simulink model "labFinal_3"  (R2018b)
settings: Solver=FixedStepDiscrete  StartTime=0.0  StopTime=10.0  FixedStep=1  RelTol=1e-3
libraries: hdlsllib x17
(part 1 of 2)
settings Model: Creator=mllax8  LastModifiedBy=mllax8

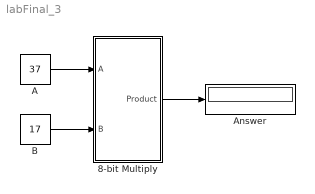
== system labFinal_3 ==
  8-bit Multiply : Subsystem
  A : Constant  Value=37  OutDataTypeStr=uint8  SampleTime=1
  Answer : Display
  B : Constant  Value=17  OutDataTypeStr=uint8  SampleTime=1
  wires:
  B/1 -> 8-bit Multiply/2(B)
  A/1 -> 8-bit Multiply/1(A)
  8-bit Multiply/1(Product) -> Answer/1

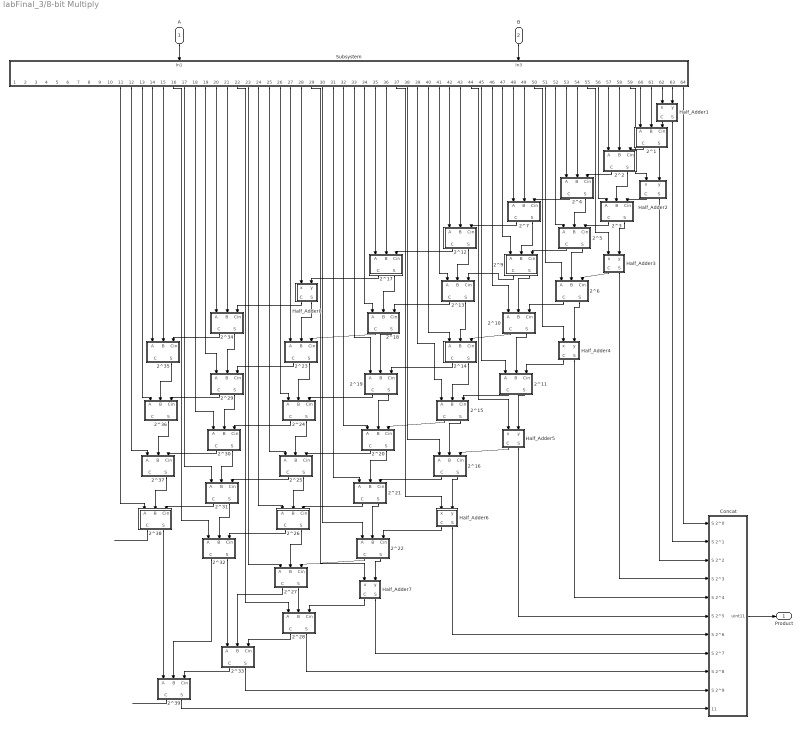
== system labFinal_3/8-bit Multiply ==
  A : Inport  OutDataTypeStr=uint8
  B : Inport  Port=2  OutDataTypeStr=uint8
  2^1 : Subsystem
  2^10 : Subsystem
  2^11 : Subsystem
  2^12 : Subsystem
  2^13 : Subsystem
  2^14 : Subsystem
  2^15 : Subsystem
  2^16 : Subsystem
  2^17 : Subsystem
  2^18 : Subsystem
  2^19 : Subsystem
  2^2 : Subsystem
  2^20 : Subsystem
  2^21 : Subsystem
  2^22 : Subsystem
  2^23 : Subsystem
  2^24 : Subsystem
  2^25 : Subsystem
  2^26 : Subsystem
  2^27 : Subsystem
  2^28 : Subsystem
  2^29 : Subsystem
  2^3 : Subsystem
  2^30 : Subsystem
  2^31 : Subsystem
  2^32 : Subsystem
  2^33 : Subsystem
  2^34 : Subsystem
  2^35 : Subsystem
  2^36 : Subsystem
  2^37 : Subsystem
  2^38 : Subsystem
  2^39 : Subsystem
  2^4 : Subsystem
  2^5 : Subsystem
  2^6 : Subsystem
  2^7 : Subsystem
  2^9 : Subsystem
  Concat : Subsystem
  Half_Adder1 : Subsystem
  Half_Adder2 : Subsystem
  Half_Adder3 : Subsystem
  Half_Adder4 : Subsystem
  Half_Adder5 : Subsystem
  Half_Adder6 : Subsystem
  Half_Adder7 : Subsystem
  Half_Adder8 : Subsystem
  Subsystem : Subsystem
  Product : Outport
  wires:
  A/1 -> Subsystem/1(In1)
  B/1 -> Subsystem/2(In3)
  Subsystem/63(A0B1) -> Half_Adder1/2(y)
  Subsystem/62(A1B0) -> Half_Adder1/1(x)
  Half_Adder1/1(C) -> 2^1/3(Cin)
  Subsystem/61(A1B1) -> 2^1/2(B)
  Subsystem/60(A0B2) -> 2^1/1(A)
  Subsystem/59(A2B0) -> Half_Adder2/1(x)
  2^1/2(S) -> Half_Adder2/2(y)
  2^1/1(C) -> 2^2/3(Cin)
  Subsystem/58(A0B3) -> 2^2/2(B)
  Subsystem/57(A1B2) -> 2^2/1(A)
  Half_Adder2/1(C) -> 2^3/3(Cin)
  2^2/2(S) -> 2^3/2(B)
  Subsystem/56(A2B1) -> 2^3/1(A)
  2^3/1(C) -> 2^5/3(Cin)
  Subsystem/55(A3B0) -> Half_Adder3/1(x)
  2^3/2(S) -> Half_Adder3/2(y)
  Subsystem/54(A0B4) -> 2^4/2(B)
  Subsystem/53(A1B3) -> 2^4/1(A)
  2^2/1(C) -> 2^4/3(Cin)
  2^4/1(C) -> 2^7/3(Cin)
  2^4/2(S) -> 2^5/2(B)
  Subsystem/52(A2B2) -> 2^5/1(A)
  2^5/1(C) -> 2^9/3(Cin)
  Half_Adder3/1(C) -> 2^6/3(Cin)
  2^5/2(S) -> 2^6/2(B)
  Subsystem/51(A3B1) -> 2^6/1(A)
  2^6/1(C) -> 2^10/3(Cin)
  2^6/2(S) -> Half_Adder4/2(y)
  Subsystem/50(A4B0) -> Half_Adder4/1(x)
  Half_Adder4/1(C) -> 2^11/3(Cin)
  Subsystem/49(A0B5) -> 2^7/2(B)
  Subsystem/48(A1B4) -> 2^7/1(A)
  Subsystem/47(A2B3) -> 2^9/1(A)
  2^9/2(S) -> 2^10/2(B)
  2^9/1(C) -> 2^13/3(Cin)
  2^7/2(S) -> 2^9/2(B)
  2^7/1(C) -> 2^12/3(Cin)
  Subsystem/46(A3B2) -> 2^10/1(A)
  2^10/1(C) -> 2^14/3(Cin)
  2^10/2(S) -> 2^11/2(B)
  Half_Adder3/2(S) -> Concat/4(S 2^3)
  Half_Adder4/2(S) -> Concat/5(S 2^4)
  2^11/1(C) -> 2^15/3(Cin)
  Subsystem/44(A5B0) -> Half_Adder5/1(x)
  2^11/2(S) -> Half_Adder5/2(y)
  Half_Adder5/2(S) -> Concat/6(S 2^5)
  Half_Adder5/1(C) -> 2^16/3(Cin)
  Subsystem/43(A0B6) -> 2^12/2(B)
  Subsystem/42(A1B5) -> 2^12/1(A)
  2^12/2(S) -> 2^13/2(B)
  Subsystem/41(A2B4) -> 2^13/1(A)
  Subsystem/45(A4B1) -> 2^11/1(A)
  2^13/1(C) -> 2^18/3(Cin)
  2^13/2(S) -> 2^14/2(B)
  Subsystem/40(A3B3) -> 2^14/1(A)
  2^14/2(S) -> 2^15/2(B)
  Subsystem/39(A4B2) -> 2^15/1(A)
  2^15/2(S) -> 2^16/2(B)
  Subsystem/38(A5B1) -> 2^16/1(A)
  2^15/1(C) -> 2^20/3(Cin)
  2^16/1(C) -> 2^21/3(Cin)
  Subsystem/37(A6B0) -> Half_Adder6/1(x)
  2^16/2(S) -> Half_Adder6/2(y)
  Half_Adder6/2(S) -> Concat/7(S 2^6)
  Half_Adder6/1(C) -> 2^22/3(Cin)
  2^17/1(C) -> Half_Adder8/2(y)
  2^12/1(C) -> 2^17/3(Cin)
  2^18/2(S) -> 2^19/2(B)
  2^21/1(C) -> 2^26/3(Cin)
  Subsystem/33(A3B4) -> 2^19/1(A)
  2^19/2(S) -> 2^20/2(B)
  Subsystem/34(A2B5) -> 2^18/1(A)
  Subsystem/32(A4B3) -> 2^20/1(A)
  2^20/2(S) -> 2^21/2(B)
  2^18/1(C) -> 2^23/3(Cin)
  Subsystem/31(A5B2) -> 2^21/1(A)
  2^17/2(S) -> 2^18/2(B)
  Subsystem/36(A0B7) -> 2^17/2(B)
  Subsystem/35(A1B6) -> 2^17/1(A)
  2^14/1(C) -> 2^19/3(Cin)
  2^21/2(S) -> 2^22/2(B)
  Subsystem/30(A6B1) -> 2^22/1(A)
  Subsystem/64(A0B0) -> Concat/1(S 2^0)
  Half_Adder2/2(S) -> Concat/3(S 2^2)
  2^22/2(S) -> Half_Adder7/2(y)
  Subsystem/29(A7B0) -> Half_Adder7/1(x)
  Subsystem/28(A1B7) -> Half_Adder8/1(x)
  Subsystem/27(A2B6) -> 2^23/1(A)
  Half_Adder8/2(S) -> 2^23/2(B)
  Half_Adder8/1(C) -> 2^34/3(Cin)
  2^19/1(C) -> 2^24/3(Cin)
  2^23/2(S) -> 2^24/2(B)
  Subsystem/26(A3B5) -> 2^24/1(A)
  2^20/1(C) -> 2^25/3(Cin)
  2^24/2(S) -> 2^25/2(B)
  Subsystem/25(A4B4) -> 2^25/1(A)
  2^24/1(C) -> 2^30/3(Cin)
  2^25/2(S) -> 2^26/2(B)
  2^25/1(C) -> 2^31/3(Cin)
  2^22/1(C) -> 2^27/3(Cin)
  Subsystem/24(A5B3) -> 2^26/1(A)
  Subsystem/23(A6B2) -> 2^27/1(A)
  Subsystem/22(A7B1) -> 2^28/1(A)
  2^26/2(S) -> 2^27/2(B)
  Half_Adder7/1(C) -> 2^28/3(Cin)
  2^27/2(S) -> 2^28/2(B)
  2^26/1(C) -> 2^32/3(Cin)
  Half_Adder7/2(S) -> Concat/8(S 2^7)
  2^28/1(C) -> 2^33/3(Cin)
  2^28/2(S) -> Concat/9(S 2^8)
  2^29/2(S) -> 2^30/2(B)
  2^30/2(S) -> 2^31/2(B)
  2^31/2(S) -> 2^32/2(B)
  Subsystem/21(A2B7) -> 2^34/2(B)
  Subsystem/20(A3B6) -> 2^34/1(A)
  2^23/1(C) -> 2^29/3(Cin)
  2^34/2(S) -> 2^29/2(B)
  Subsystem/19(A4B5) -> 2^29/1(A)
  Subsystem/18(A5B4) -> 2^30/1(A)
  Subsystem/17(A6B3) -> 2^31/1(A)
  Subsystem/16(A7B2) -> 2^32/1(A)
  2^32/2(S) -> 2^33/1(A)
  2^27/1(C) -> 2^33/2(B)
  2^33/2(S) -> Concat/10(S 2^9)
  2^32/1(C) -> 2^39/2(B)
  2^33/1(C) -> 2^39/3(Cin)
  2^34/1(C) -> 2^35/3(Cin)
  Subsystem/15(A3B7) -> 2^35/2(B)
  Subsystem/14(A4B6) -> 2^35/1(A)
  2^35/2(S) -> 2^36/2(B)
  2^29/1(C) -> 2^36/3(Cin)
  2^30/1(C) -> 2^37/3(Cin)
  2^36/2(S) -> 2^37/2(B)
  Subsystem/13(A5B5) -> 2^36/1(A)
  Subsystem/12(A6B4) -> 2^37/1(A)
  Subsystem/11(A7B3) -> 2^38/1(A)
  2^31/1(C) -> 2^38/3(Cin)
  2^37/2(S) -> 2^38/2(B)
  2^38/2(S) -> 2^39/1(A)
  2^38/1(C) -> ?
  2^39/1(C) -> ?
  2^39/2(S) -> Concat/11(S 2^10)
  Half_Adder1/2(S) -> Concat/2(S 2^1)
  Concat/1(uint11) -> Product/1

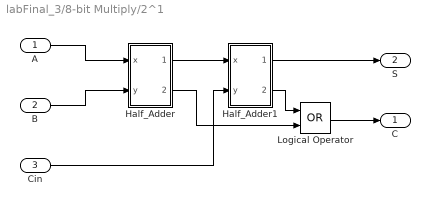
== system labFinal_3/8-bit Multiply/2^1 ==
  A : Inport
  B : Inport  Port=2
  Cin : Inport  Port=3
  Half_Adder : Subsystem
  Half_Adder1 : Subsystem
  Logical Operator : Logic  Operator=OR  AllPortsSameDT=off  OutDataTypeStr=boolean
  C : Outport
  S : Outport  Port=2
  wires:
  Half_Adder1/1(Sum) -> S/1
  Cin/1 -> Half_Adder1/2(y)
  Logical Operator/1 -> C/1
  Half_Adder1/2(Carry) -> Logical Operator/1
  A/1 -> Half_Adder/1(x)
  B/1 -> Half_Adder/2(y)
  Half_Adder/2(Carry) -> Logical Operator/2
  Half_Adder/1(Sum) -> Half_Adder1/1(x)

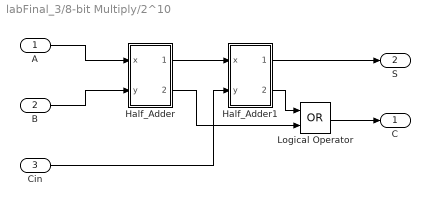
== system labFinal_3/8-bit Multiply/2^10 ==
  A : Inport
  B : Inport  Port=2
  Cin : Inport  Port=3
  Half_Adder : Subsystem
  Half_Adder1 : Subsystem
  Logical Operator : Logic  Operator=OR  AllPortsSameDT=off  OutDataTypeStr=boolean
  C : Outport
  S : Outport  Port=2
  wires:
  Half_Adder1/1(Sum) -> S/1
  Cin/1 -> Half_Adder1/2(y)
  Logical Operator/1 -> C/1
  Half_Adder1/2(Carry) -> Logical Operator/1
  A/1 -> Half_Adder/1(x)
  B/1 -> Half_Adder/2(y)
  Half_Adder/2(Carry) -> Logical Operator/2
  Half_Adder/1(Sum) -> Half_Adder1/1(x)

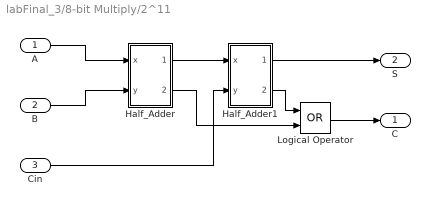
== system labFinal_3/8-bit Multiply/2^11 ==
  A : Inport
  B : Inport  Port=2
  Cin : Inport  Port=3
  Half_Adder : Subsystem
  Half_Adder1 : Subsystem
  Logical Operator : Logic  Operator=OR  AllPortsSameDT=off  OutDataTypeStr=boolean
  C : Outport
  S : Outport  Port=2
  wires:
  Half_Adder1/1(Sum) -> S/1
  Cin/1 -> Half_Adder1/2(y)
  Logical Operator/1 -> C/1
  Half_Adder1/2(Carry) -> Logical Operator/1
  A/1 -> Half_Adder/1(x)
  B/1 -> Half_Adder/2(y)
  Half_Adder/2(Carry) -> Logical Operator/2
  Half_Adder/1(Sum) -> Half_Adder1/1(x)

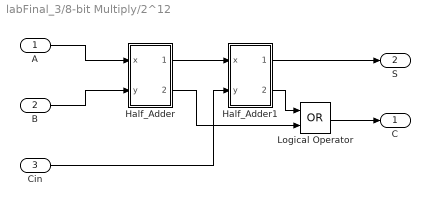
== system labFinal_3/8-bit Multiply/2^12 ==
  A : Inport
  B : Inport  Port=2
  Cin : Inport  Port=3
  Half_Adder : Subsystem
  Half_Adder1 : Subsystem
  Logical Operator : Logic  Operator=OR  AllPortsSameDT=off  OutDataTypeStr=boolean
  C : Outport
  S : Outport  Port=2
  wires:
  Half_Adder1/1(Sum) -> S/1
  Cin/1 -> Half_Adder1/2(y)
  Logical Operator/1 -> C/1
  Half_Adder1/2(Carry) -> Logical Operator/1
  A/1 -> Half_Adder/1(x)
  B/1 -> Half_Adder/2(y)
  Half_Adder/2(Carry) -> Logical Operator/2
  Half_Adder/1(Sum) -> Half_Adder1/1(x)

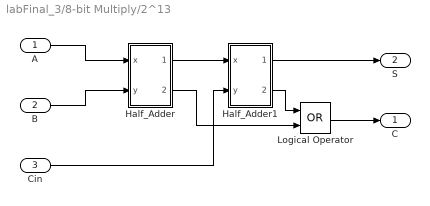
== system labFinal_3/8-bit Multiply/2^13 ==
  A : Inport
  B : Inport  Port=2
  Cin : Inport  Port=3
  Half_Adder : Subsystem
  Half_Adder1 : Subsystem
  Logical Operator : Logic  Operator=OR  AllPortsSameDT=off  OutDataTypeStr=boolean
  C : Outport
  S : Outport  Port=2
  wires:
  Half_Adder1/1(Sum) -> S/1
  Cin/1 -> Half_Adder1/2(y)
  Logical Operator/1 -> C/1
  Half_Adder1/2(Carry) -> Logical Operator/1
  A/1 -> Half_Adder/1(x)
  B/1 -> Half_Adder/2(y)
  Half_Adder/2(Carry) -> Logical Operator/2
  Half_Adder/1(Sum) -> Half_Adder1/1(x)

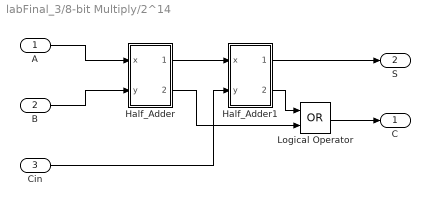
== system labFinal_3/8-bit Multiply/2^14 ==
  A : Inport
  B : Inport  Port=2
  Cin : Inport  Port=3
  Half_Adder : Subsystem
  Half_Adder1 : Subsystem
  Logical Operator : Logic  Operator=OR  AllPortsSameDT=off  OutDataTypeStr=boolean
  C : Outport
  S : Outport  Port=2
  wires:
  Half_Adder1/1(Sum) -> S/1
  Cin/1 -> Half_Adder1/2(y)
  Logical Operator/1 -> C/1
  Half_Adder1/2(Carry) -> Logical Operator/1
  A/1 -> Half_Adder/1(x)
  B/1 -> Half_Adder/2(y)
  Half_Adder/2(Carry) -> Logical Operator/2
  Half_Adder/1(Sum) -> Half_Adder1/1(x)

== system labFinal_3/8-bit Multiply/2^15 ==
  A : Inport
  B : Inport  Port=2
  Cin : Inport  Port=3
  Half_Adder : Subsystem
  Half_Adder1 : Subsystem
  Logical Operator : Logic  Operator=OR  AllPortsSameDT=off  OutDataTypeStr=boolean
  C : Outport
  S : Outport  Port=2
  wires:
  Half_Adder1/1(Sum) -> S/1
  Cin/1 -> Half_Adder1/2(y)
  Logical Operator/1 -> C/1
  Half_Adder1/2(Carry) -> Logical Operator/1
  A/1 -> Half_Adder/1(x)
  B/1 -> Half_Adder/2(y)
  Half_Adder/2(Carry) -> Logical Operator/2
  Half_Adder/1(Sum) -> Half_Adder1/1(x)

== system labFinal_3/8-bit Multiply/2^16 ==
  A : Inport
  B : Inport  Port=2
  Cin : Inport  Port=3
  Half_Adder : Subsystem
  Half_Adder1 : Subsystem
  Logical Operator : Logic  Operator=OR  AllPortsSameDT=off  OutDataTypeStr=boolean
  C : Outport
  S : Outport  Port=2
  wires:
  Half_Adder1/1(Sum) -> S/1
  Cin/1 -> Half_Adder1/2(y)
  Logical Operator/1 -> C/1
  Half_Adder1/2(Carry) -> Logical Operator/1
  A/1 -> Half_Adder/1(x)
  B/1 -> Half_Adder/2(y)
  Half_Adder/2(Carry) -> Logical Operator/2
  Half_Adder/1(Sum) -> Half_Adder1/1(x)

== system labFinal_3/8-bit Multiply/2^17 ==
  A : Inport
  B : Inport  Port=2
  Cin : Inport  Port=3
  Half_Adder : Subsystem
  Half_Adder1 : Subsystem
  Logical Operator : Logic  Operator=OR  AllPortsSameDT=off  OutDataTypeStr=boolean
  C : Outport
  S : Outport  Port=2
  wires:
  Half_Adder1/1(Sum) -> S/1
  Cin/1 -> Half_Adder1/2(y)
  Logical Operator/1 -> C/1
  Half_Adder1/2(Carry) -> Logical Operator/1
  A/1 -> Half_Adder/1(x)
  B/1 -> Half_Adder/2(y)
  Half_Adder/2(Carry) -> Logical Operator/2
  Half_Adder/1(Sum) -> Half_Adder1/1(x)

== system labFinal_3/8-bit Multiply/2^18 ==
  A : Inport
  B : Inport  Port=2
  Cin : Inport  Port=3
  Half_Adder : Subsystem
  Half_Adder1 : Subsystem
  Logical Operator : Logic  Operator=OR  AllPortsSameDT=off  OutDataTypeStr=boolean
  C : Outport
  S : Outport  Port=2
  wires:
  Half_Adder1/1(Sum) -> S/1
  Cin/1 -> Half_Adder1/2(y)
  Logical Operator/1 -> C/1
  Half_Adder1/2(Carry) -> Logical Operator/1
  A/1 -> Half_Adder/1(x)
  B/1 -> Half_Adder/2(y)
  Half_Adder/2(Carry) -> Logical Operator/2
  Half_Adder/1(Sum) -> Half_Adder1/1(x)

== system labFinal_3/8-bit Multiply/2^19 ==
  A : Inport
  B : Inport  Port=2
  Cin : Inport  Port=3
  Half_Adder : Subsystem
  Half_Adder1 : Subsystem
  Logical Operator : Logic  Operator=OR  AllPortsSameDT=off  OutDataTypeStr=boolean
  C : Outport
  S : Outport  Port=2
  wires:
  Half_Adder1/1(Sum) -> S/1
  Cin/1 -> Half_Adder1/2(y)
  Logical Operator/1 -> C/1
  Half_Adder1/2(Carry) -> Logical Operator/1
  A/1 -> Half_Adder/1(x)
  B/1 -> Half_Adder/2(y)
  Half_Adder/2(Carry) -> Logical Operator/2
  Half_Adder/1(Sum) -> Half_Adder1/1(x)

== system labFinal_3/8-bit Multiply/2^2 ==
  A : Inport
  B : Inport  Port=2
  Cin : Inport  Port=3
  Half_Adder : Subsystem
  Half_Adder1 : Subsystem
  Logical Operator : Logic  Operator=OR  AllPortsSameDT=off  OutDataTypeStr=boolean
  C : Outport
  S : Outport  Port=2
  wires:
  Half_Adder1/1(Sum) -> S/1
  Cin/1 -> Half_Adder1/2(y)
  Logical Operator/1 -> C/1
  Half_Adder1/2(Carry) -> Logical Operator/1
  A/1 -> Half_Adder/1(x)
  B/1 -> Half_Adder/2(y)
  Half_Adder/2(Carry) -> Logical Operator/2
  Half_Adder/1(Sum) -> Half_Adder1/1(x)

== system labFinal_3/8-bit Multiply/2^20 ==
  A : Inport
  B : Inport  Port=2
  Cin : Inport  Port=3
  Half_Adder : Subsystem
  Half_Adder1 : Subsystem
  Logical Operator : Logic  Operator=OR  AllPortsSameDT=off  OutDataTypeStr=boolean
  C : Outport
  S : Outport  Port=2
  wires:
  Half_Adder1/1(Sum) -> S/1
  Cin/1 -> Half_Adder1/2(y)
  Logical Operator/1 -> C/1
  Half_Adder1/2(Carry) -> Logical Operator/1
  A/1 -> Half_Adder/1(x)
  B/1 -> Half_Adder/2(y)
  Half_Adder/2(Carry) -> Logical Operator/2
  Half_Adder/1(Sum) -> Half_Adder1/1(x)

== system labFinal_3/8-bit Multiply/2^21 ==
  A : Inport
  B : Inport  Port=2
  Cin : Inport  Port=3
  Half_Adder : Subsystem
  Half_Adder1 : Subsystem
  Logical Operator : Logic  Operator=OR  AllPortsSameDT=off  OutDataTypeStr=boolean
  C : Outport
  S : Outport  Port=2
  wires:
  Half_Adder1/1(Sum) -> S/1
  Cin/1 -> Half_Adder1/2(y)
  Logical Operator/1 -> C/1
  Half_Adder1/2(Carry) -> Logical Operator/1
  A/1 -> Half_Adder/1(x)
  B/1 -> Half_Adder/2(y)
  Half_Adder/2(Carry) -> Logical Operator/2
  Half_Adder/1(Sum) -> Half_Adder1/1(x)

== system labFinal_3/8-bit Multiply/2^22 ==
  A : Inport
  B : Inport  Port=2
  Cin : Inport  Port=3
  Half_Adder : Subsystem
  Half_Adder1 : Subsystem
  Logical Operator : Logic  Operator=OR  AllPortsSameDT=off  OutDataTypeStr=boolean
  C : Outport
  S : Outport  Port=2
  wires:
  Half_Adder1/1(Sum) -> S/1
  Cin/1 -> Half_Adder1/2(y)
  Logical Operator/1 -> C/1
  Half_Adder1/2(Carry) -> Logical Operator/1
  A/1 -> Half_Adder/1(x)
  B/1 -> Half_Adder/2(y)
  Half_Adder/2(Carry) -> Logical Operator/2
  Half_Adder/1(Sum) -> Half_Adder1/1(x)

== system labFinal_3/8-bit Multiply/2^23 ==
  A : Inport
  B : Inport  Port=2
  Cin : Inport  Port=3
  Half_Adder : Subsystem
  Half_Adder1 : Subsystem
  Logical Operator : Logic  Operator=OR  AllPortsSameDT=off  OutDataTypeStr=boolean
  C : Outport
  S : Outport  Port=2
  wires:
  Half_Adder1/1(Sum) -> S/1
  Cin/1 -> Half_Adder1/2(y)
  Logical Operator/1 -> C/1
  Half_Adder1/2(Carry) -> Logical Operator/1
  A/1 -> Half_Adder/1(x)
  B/1 -> Half_Adder/2(y)
  Half_Adder/2(Carry) -> Logical Operator/2
  Half_Adder/1(Sum) -> Half_Adder1/1(x)

== system labFinal_3/8-bit Multiply/2^24 ==
  A : Inport
  B : Inport  Port=2
  Cin : Inport  Port=3
  Half_Adder : Subsystem
  Half_Adder1 : Subsystem
  Logical Operator : Logic  Operator=OR  AllPortsSameDT=off  OutDataTypeStr=boolean
  C : Outport
  S : Outport  Port=2
  wires:
  Half_Adder1/1(Sum) -> S/1
  Cin/1 -> Half_Adder1/2(y)
  Logical Operator/1 -> C/1
  Half_Adder1/2(Carry) -> Logical Operator/1
  A/1 -> Half_Adder/1(x)
  B/1 -> Half_Adder/2(y)
  Half_Adder/2(Carry) -> Logical Operator/2
  Half_Adder/1(Sum) -> Half_Adder1/1(x)

== system labFinal_3/8-bit Multiply/2^25 ==
  A : Inport
  B : Inport  Port=2
  Cin : Inport  Port=3
  Half_Adder : Subsystem
  Half_Adder1 : Subsystem
  Logical Operator : Logic  Operator=OR  AllPortsSameDT=off  OutDataTypeStr=boolean
  C : Outport
  S : Outport  Port=2
  wires:
  Half_Adder1/1(Sum) -> S/1
  Cin/1 -> Half_Adder1/2(y)
  Logical Operator/1 -> C/1
  Half_Adder1/2(Carry) -> Logical Operator/1
  A/1 -> Half_Adder/1(x)
  B/1 -> Half_Adder/2(y)
  Half_Adder/2(Carry) -> Logical Operator/2
  Half_Adder/1(Sum) -> Half_Adder1/1(x)

== system labFinal_3/8-bit Multiply/2^26 ==
  A : Inport
  B : Inport  Port=2
  Cin : Inport  Port=3
  Half_Adder : Subsystem
  Half_Adder1 : Subsystem
  Logical Operator : Logic  Operator=OR  AllPortsSameDT=off  OutDataTypeStr=boolean
  C : Outport
  S : Outport  Port=2
  wires:
  Half_Adder1/1(Sum) -> S/1
  Cin/1 -> Half_Adder1/2(y)
  Logical Operator/1 -> C/1
  Half_Adder1/2(Carry) -> Logical Operator/1
  A/1 -> Half_Adder/1(x)
  B/1 -> Half_Adder/2(y)
  Half_Adder/2(Carry) -> Logical Operator/2
  Half_Adder/1(Sum) -> Half_Adder1/1(x)

== system labFinal_3/8-bit Multiply/2^27 ==
  A : Inport
  B : Inport  Port=2
  Cin : Inport  Port=3
  Half_Adder : Subsystem
  Half_Adder1 : Subsystem
  Logical Operator : Logic  Operator=OR  AllPortsSameDT=off  OutDataTypeStr=boolean
  C : Outport
  S : Outport  Port=2
  wires:
  Half_Adder1/1(Sum) -> S/1
  Cin/1 -> Half_Adder1/2(y)
  Logical Operator/1 -> C/1
  Half_Adder1/2(Carry) -> Logical Operator/1
  A/1 -> Half_Adder/1(x)
  B/1 -> Half_Adder/2(y)
  Half_Adder/2(Carry) -> Logical Operator/2
  Half_Adder/1(Sum) -> Half_Adder1/1(x)

== system labFinal_3/8-bit Multiply/2^28 ==
  A : Inport
  B : Inport  Port=2
  Cin : Inport  Port=3
  Half_Adder : Subsystem
  Half_Adder1 : Subsystem
  Logical Operator : Logic  Operator=OR  AllPortsSameDT=off  OutDataTypeStr=boolean
  C : Outport
  S : Outport  Port=2
  wires:
  Half_Adder1/1(Sum) -> S/1
  Cin/1 -> Half_Adder1/2(y)
  Logical Operator/1 -> C/1
  Half_Adder1/2(Carry) -> Logical Operator/1
  A/1 -> Half_Adder/1(x)
  B/1 -> Half_Adder/2(y)
  Half_Adder/2(Carry) -> Logical Operator/2
  Half_Adder/1(Sum) -> Half_Adder1/1(x)

== system labFinal_3/8-bit Multiply/2^29 ==
  A : Inport
  B : Inport  Port=2
  Cin : Inport  Port=3
  Half_Adder : Subsystem
  Half_Adder1 : Subsystem
  Logical Operator : Logic  Operator=OR  AllPortsSameDT=off  OutDataTypeStr=boolean
  C : Outport
  S : Outport  Port=2
  wires:
  Half_Adder1/1(Sum) -> S/1
  Cin/1 -> Half_Adder1/2(y)
  Logical Operator/1 -> C/1
  Half_Adder1/2(Carry) -> Logical Operator/1
  A/1 -> Half_Adder/1(x)
  B/1 -> Half_Adder/2(y)
  Half_Adder/2(Carry) -> Logical Operator/2
  Half_Adder/1(Sum) -> Half_Adder1/1(x)

== system labFinal_3/8-bit Multiply/2^3 ==
  A : Inport
  B : Inport  Port=2
  Cin : Inport  Port=3
  Half_Adder : Subsystem
  Half_Adder1 : Subsystem
  Logical Operator : Logic  Operator=OR  AllPortsSameDT=off  OutDataTypeStr=boolean
  C : Outport
  S : Outport  Port=2
  wires:
  Half_Adder1/1(Sum) -> S/1
  Cin/1 -> Half_Adder1/2(y)
  Logical Operator/1 -> C/1
  Half_Adder1/2(Carry) -> Logical Operator/1
  A/1 -> Half_Adder/1(x)
  B/1 -> Half_Adder/2(y)
  Half_Adder/2(Carry) -> Logical Operator/2
  Half_Adder/1(Sum) -> Half_Adder1/1(x)

== system labFinal_3/8-bit Multiply/2^30 ==
  A : Inport
  B : Inport  Port=2
  Cin : Inport  Port=3
  Half_Adder : Subsystem
  Half_Adder1 : Subsystem
  Logical Operator : Logic  Operator=OR  AllPortsSameDT=off  OutDataTypeStr=boolean
  C : Outport
  S : Outport  Port=2
  wires:
  Half_Adder1/1(Sum) -> S/1
  Cin/1 -> Half_Adder1/2(y)
  Logical Operator/1 -> C/1
  Half_Adder1/2(Carry) -> Logical Operator/1
  A/1 -> Half_Adder/1(x)
  B/1 -> Half_Adder/2(y)
  Half_Adder/2(Carry) -> Logical Operator/2
  Half_Adder/1(Sum) -> Half_Adder1/1(x)

== system labFinal_3/8-bit Multiply/2^31 ==
  A : Inport
  B : Inport  Port=2
  Cin : Inport  Port=3
  Half_Adder : Subsystem
  Half_Adder1 : Subsystem
  Logical Operator : Logic  Operator=OR  AllPortsSameDT=off  OutDataTypeStr=boolean
  C : Outport
  S : Outport  Port=2
  wires:
  Half_Adder1/1(Sum) -> S/1
  Cin/1 -> Half_Adder1/2(y)
  Logical Operator/1 -> C/1
  Half_Adder1/2(Carry) -> Logical Operator/1
  A/1 -> Half_Adder/1(x)
  B/1 -> Half_Adder/2(y)
  Half_Adder/2(Carry) -> Logical Operator/2
  Half_Adder/1(Sum) -> Half_Adder1/1(x)

== system labFinal_3/8-bit Multiply/2^32 ==
  A : Inport
  B : Inport  Port=2
  Cin : Inport  Port=3
  Half_Adder : Subsystem
  Half_Adder1 : Subsystem
  Logical Operator : Logic  Operator=OR  AllPortsSameDT=off  OutDataTypeStr=boolean
  C : Outport
  S : Outport  Port=2
  wires:
  Half_Adder1/1(Sum) -> S/1
  Cin/1 -> Half_Adder1/2(y)
  Logical Operator/1 -> C/1
  Half_Adder1/2(Carry) -> Logical Operator/1
  A/1 -> Half_Adder/1(x)
  B/1 -> Half_Adder/2(y)
  Half_Adder/2(Carry) -> Logical Operator/2
  Half_Adder/1(Sum) -> Half_Adder1/1(x)

== system labFinal_3/8-bit Multiply/2^33 ==
  A : Inport
  B : Inport  Port=2
  Cin : Inport  Port=3
  Half_Adder : Subsystem
  Half_Adder1 : Subsystem
  Logical Operator : Logic  Operator=OR  AllPortsSameDT=off  OutDataTypeStr=boolean
  C : Outport
  S : Outport  Port=2
  wires:
  Half_Adder1/1(Sum) -> S/1
  Cin/1 -> Half_Adder1/2(y)
  Logical Operator/1 -> C/1
  Half_Adder1/2(Carry) -> Logical Operator/1
  A/1 -> Half_Adder/1(x)
  B/1 -> Half_Adder/2(y)
  Half_Adder/2(Carry) -> Logical Operator/2
  Half_Adder/1(Sum) -> Half_Adder1/1(x)

== system labFinal_3/8-bit Multiply/2^34 ==
  A : Inport
  B : Inport  Port=2
  Cin : Inport  Port=3
  Half_Adder : Subsystem
  Half_Adder1 : Subsystem
  Logical Operator : Logic  Operator=OR  AllPortsSameDT=off  OutDataTypeStr=boolean
  C : Outport
  S : Outport  Port=2
  wires:
  Half_Adder1/1(Sum) -> S/1
  Cin/1 -> Half_Adder1/2(y)
  Logical Operator/1 -> C/1
  Half_Adder1/2(Carry) -> Logical Operator/1
  A/1 -> Half_Adder/1(x)
  B/1 -> Half_Adder/2(y)
  Half_Adder/2(Carry) -> Logical Operator/2
  Half_Adder/1(Sum) -> Half_Adder1/1(x)

== system labFinal_3/8-bit Multiply/2^35 ==
  A : Inport
  B : Inport  Port=2
  Cin : Inport  Port=3
  Half_Adder : Subsystem
  Half_Adder1 : Subsystem
  Logical Operator : Logic  Operator=OR  AllPortsSameDT=off  OutDataTypeStr=boolean
  C : Outport
  S : Outport  Port=2
  wires:
  Half_Adder1/1(Sum) -> S/1
  Cin/1 -> Half_Adder1/2(y)
  Logical Operator/1 -> C/1
  Half_Adder1/2(Carry) -> Logical Operator/1
  A/1 -> Half_Adder/1(x)
  B/1 -> Half_Adder/2(y)
  Half_Adder/2(Carry) -> Logical Operator/2
  Half_Adder/1(Sum) -> Half_Adder1/1(x)

== system labFinal_3/8-bit Multiply/2^36 ==
  A : Inport
  B : Inport  Port=2
  Cin : Inport  Port=3
  Half_Adder : Subsystem
  Half_Adder1 : Subsystem
  Logical Operator : Logic  Operator=OR  AllPortsSameDT=off  OutDataTypeStr=boolean
  C : Outport
  S : Outport  Port=2
  wires:
  Half_Adder1/1(Sum) -> S/1
  Cin/1 -> Half_Adder1/2(y)
  Logical Operator/1 -> C/1
  Half_Adder1/2(Carry) -> Logical Operator/1
  A/1 -> Half_Adder/1(x)
  B/1 -> Half_Adder/2(y)
  Half_Adder/2(Carry) -> Logical Operator/2
  Half_Adder/1(Sum) -> Half_Adder1/1(x)

== system labFinal_3/8-bit Multiply/2^37 ==
  A : Inport
  B : Inport  Port=2
  Cin : Inport  Port=3
  Half_Adder : Subsystem
  Half_Adder1 : Subsystem
  Logical Operator : Logic  Operator=OR  AllPortsSameDT=off  OutDataTypeStr=boolean
  C : Outport
  S : Outport  Port=2
  wires:
  Half_Adder1/1(Sum) -> S/1
  Cin/1 -> Half_Adder1/2(y)
  Logical Operator/1 -> C/1
  Half_Adder1/2(Carry) -> Logical Operator/1
  A/1 -> Half_Adder/1(x)
  B/1 -> Half_Adder/2(y)
  Half_Adder/2(Carry) -> Logical Operator/2
  Half_Adder/1(Sum) -> Half_Adder1/1(x)

== system labFinal_3/8-bit Multiply/2^38 ==
  A : Inport
  B : Inport  Port=2
  Cin : Inport  Port=3
  Half_Adder : Subsystem
  Half_Adder1 : Subsystem
  Logical Operator : Logic  Operator=OR  AllPortsSameDT=off  OutDataTypeStr=boolean
  C : Outport
  S : Outport  Port=2
  wires:
  Half_Adder1/1(Sum) -> S/1
  Cin/1 -> Half_Adder1/2(y)
  Logical Operator/1 -> C/1
  Half_Adder1/2(Carry) -> Logical Operator/1
  A/1 -> Half_Adder/1(x)
  B/1 -> Half_Adder/2(y)
  Half_Adder/2(Carry) -> Logical Operator/2
  Half_Adder/1(Sum) -> Half_Adder1/1(x)

== system labFinal_3/8-bit Multiply/2^39 ==
  A : Inport
  B : Inport  Port=2
  Cin : Inport  Port=3
  Half_Adder : Subsystem
  Half_Adder1 : Subsystem
  Logical Operator : Logic  Operator=OR  AllPortsSameDT=off  OutDataTypeStr=boolean
  C : Outport
  S : Outport  Port=2
  wires:
  Half_Adder1/1(Sum) -> S/1
  Cin/1 -> Half_Adder1/2(y)
  Logical Operator/1 -> C/1
  Half_Adder1/2(Carry) -> Logical Operator/1
  A/1 -> Half_Adder/1(x)
  B/1 -> Half_Adder/2(y)
  Half_Adder/2(Carry) -> Logical Operator/2
  Half_Adder/1(Sum) -> Half_Adder1/1(x)

== system labFinal_3/8-bit Multiply/2^4 ==
  A : Inport
  B : Inport  Port=2
  Cin : Inport  Port=3
  Half_Adder : Subsystem
  Half_Adder1 : Subsystem
  Logical Operator : Logic  Operator=OR  AllPortsSameDT=off  OutDataTypeStr=boolean
  C : Outport
  S : Outport  Port=2
  wires:
  Half_Adder1/1(Sum) -> S/1
  Cin/1 -> Half_Adder1/2(y)
  Logical Operator/1 -> C/1
  Half_Adder1/2(Carry) -> Logical Operator/1
  A/1 -> Half_Adder/1(x)
  B/1 -> Half_Adder/2(y)
  Half_Adder/2(Carry) -> Logical Operator/2
  Half_Adder/1(Sum) -> Half_Adder1/1(x)

== system labFinal_3/8-bit Multiply/2^5 ==
  A : Inport
  B : Inport  Port=2
  Cin : Inport  Port=3
  Half_Adder : Subsystem
  Half_Adder1 : Subsystem
  Logical Operator : Logic  Operator=OR  AllPortsSameDT=off  OutDataTypeStr=boolean
  C : Outport
  S : Outport  Port=2
  wires:
  Half_Adder1/1(Sum) -> S/1
  Cin/1 -> Half_Adder1/2(y)
  Logical Operator/1 -> C/1
  Half_Adder1/2(Carry) -> Logical Operator/1
  A/1 -> Half_Adder/1(x)
  B/1 -> Half_Adder/2(y)
  Half_Adder/2(Carry) -> Logical Operator/2
  Half_Adder/1(Sum) -> Half_Adder1/1(x)

== system labFinal_3/8-bit Multiply/2^6 ==
  A : Inport
  B : Inport  Port=2
  Cin : Inport  Port=3
  Half_Adder : Subsystem
  Half_Adder1 : Subsystem
  Logical Operator : Logic  Operator=OR  AllPortsSameDT=off  OutDataTypeStr=boolean
  C : Outport
  S : Outport  Port=2
  wires:
  Half_Adder1/1(Sum) -> S/1
  Cin/1 -> Half_Adder1/2(y)
  Logical Operator/1 -> C/1
  Half_Adder1/2(Carry) -> Logical Operator/1
  A/1 -> Half_Adder/1(x)
  B/1 -> Half_Adder/2(y)
  Half_Adder/2(Carry) -> Logical Operator/2
  Half_Adder/1(Sum) -> Half_Adder1/1(x)

== system labFinal_3/8-bit Multiply/2^7 ==
  A : Inport
  B : Inport  Port=2
  Cin : Inport  Port=3
  Half_Adder : Subsystem
  Half_Adder1 : Subsystem
  Logical Operator : Logic  Operator=OR  AllPortsSameDT=off  OutDataTypeStr=boolean
  C : Outport
  S : Outport  Port=2
  wires:
  Half_Adder1/1(Sum) -> S/1
  Cin/1 -> Half_Adder1/2(y)
  Logical Operator/1 -> C/1
  Half_Adder1/2(Carry) -> Logical Operator/1
  A/1 -> Half_Adder/1(x)
  B/1 -> Half_Adder/2(y)
  Half_Adder/2(Carry) -> Logical Operator/2
  Half_Adder/1(Sum) -> Half_Adder1/1(x)

== system labFinal_3/8-bit Multiply/2^9 ==
  A : Inport
  B : Inport  Port=2
  Cin : Inport  Port=3
  Half_Adder : Subsystem
  Half_Adder1 : Subsystem
  Logical Operator : Logic  Operator=OR  AllPortsSameDT=off  OutDataTypeStr=boolean
  C : Outport
  S : Outport  Port=2
  wires:
  Half_Adder1/1(Sum) -> S/1
  Cin/1 -> Half_Adder1/2(y)
  Logical Operator/1 -> C/1
  Half_Adder1/2(Carry) -> Logical Operator/1
  A/1 -> Half_Adder/1(x)
  B/1 -> Half_Adder/2(y)
  Half_Adder/2(Carry) -> Logical Operator/2
  Half_Adder/1(Sum) -> Half_Adder1/1(x)

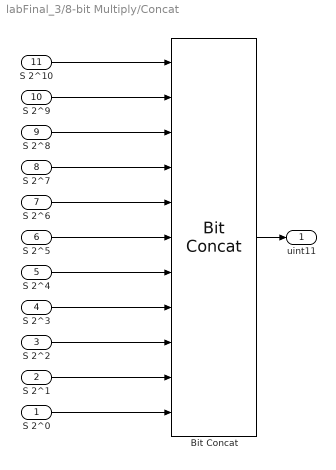
== system labFinal_3/8-bit Multiply/Concat ==
  S 2^0 : Inport
  S 2^1 : Inport  Port=2
  S 2^2 : Inport  Port=3
  S 2^3 : Inport  Port=4
  S 2^4 : Inport  Port=5
  S 2^5 : Inport  Port=6
  S 2^6 : Inport  Port=7
  S 2^7 : Inport  Port=8
  S 2^8 : Inport  Port=9
  S 2^9 : Inport  Port=10
  S 2^10 : Inport  Port=11
  Bit Concat : hdlsllib/Logic and Bit Operations/Bit Concat  numInputs=11
      settings: SourceProductName=HDL Coder  SourceProductBaseCode=HD
  uint11 : Outport
  wires:
  Bit Concat/1 -> uint11/1
  S 2^0/1 -> Bit Concat/11
  S 2^1/1 -> Bit Concat/10
  S 2^2/1 -> Bit Concat/9
  S 2^3/1 -> Bit Concat/8
  S 2^4/1 -> Bit Concat/7
  S 2^5/1 -> Bit Concat/6
  S 2^6/1 -> Bit Concat/5
  S 2^7/1 -> Bit Concat/4
  S 2^10/1 -> Bit Concat/1
  S 2^9/1 -> Bit Concat/2
  S 2^8/1 -> Bit Concat/3

== system labFinal_3/8-bit Multiply/Half_Adder1 ==
  x : Inport
  y : Inport  Port=2
  Calc Carry : Logic  AllPortsSameDT=off  OutDataTypeStr=boolean
  Calc Sum : Logic  Operator=XOR  AllPortsSameDT=off  OutDataTypeStr=boolean
  C : Outport
  S : Outport  Port=2
  wires:
  Calc Carry/1 -> C/1
  x/1 -> Calc Carry/1, Calc Sum/1
  Calc Sum/1 -> S/1
  y/1 -> Calc Sum/2, Calc Carry/2

== system labFinal_3/8-bit Multiply/Half_Adder2 ==
  x : Inport
  y : Inport  Port=2
  Calc Carry : Logic  AllPortsSameDT=off  OutDataTypeStr=boolean
  Calc Sum : Logic  Operator=XOR  AllPortsSameDT=off  OutDataTypeStr=boolean
  C : Outport
  S : Outport  Port=2
  wires:
  Calc Carry/1 -> C/1
  x/1 -> Calc Carry/1, Calc Sum/1
  Calc Sum/1 -> S/1
  y/1 -> Calc Sum/2, Calc Carry/2

== system labFinal_3/8-bit Multiply/Half_Adder3 ==
  x : Inport
  y : Inport  Port=2
  Calc Carry : Logic  AllPortsSameDT=off  OutDataTypeStr=boolean
  Calc Sum : Logic  Operator=XOR  AllPortsSameDT=off  OutDataTypeStr=boolean
  C : Outport
  S : Outport  Port=2
  wires:
  Calc Carry/1 -> C/1
  x/1 -> Calc Carry/1, Calc Sum/1
  Calc Sum/1 -> S/1
  y/1 -> Calc Sum/2, Calc Carry/2

== system labFinal_3/8-bit Multiply/Half_Adder4 ==
  x : Inport
  y : Inport  Port=2
  Calc Carry : Logic  AllPortsSameDT=off  OutDataTypeStr=boolean
  Calc Sum : Logic  Operator=XOR  AllPortsSameDT=off  OutDataTypeStr=boolean
  C : Outport
  S : Outport  Port=2
  wires:
  Calc Carry/1 -> C/1
  x/1 -> Calc Carry/1, Calc Sum/1
  Calc Sum/1 -> S/1
  y/1 -> Calc Sum/2, Calc Carry/2

== system labFinal_3/8-bit Multiply/Half_Adder5 ==
  x : Inport
  y : Inport  Port=2
  Calc Carry : Logic  AllPortsSameDT=off  OutDataTypeStr=boolean
  Calc Sum : Logic  Operator=XOR  AllPortsSameDT=off  OutDataTypeStr=boolean
  C : Outport
  S : Outport  Port=2
  wires:
  Calc Carry/1 -> C/1
  x/1 -> Calc Carry/1, Calc Sum/1
  Calc Sum/1 -> S/1
  y/1 -> Calc Sum/2, Calc Carry/2

== system labFinal_3/8-bit Multiply/Half_Adder6 ==
  x : Inport
  y : Inport  Port=2
  Calc Carry : Logic  AllPortsSameDT=off  OutDataTypeStr=boolean
  Calc Sum : Logic  Operator=XOR  AllPortsSameDT=off  OutDataTypeStr=boolean
  C : Outport
  S : Outport  Port=2
  wires:
  Calc Carry/1 -> C/1
  x/1 -> Calc Carry/1, Calc Sum/1
  Calc Sum/1 -> S/1
  y/1 -> Calc Sum/2, Calc Carry/2

== system labFinal_3/8-bit Multiply/Half_Adder7 ==
  x : Inport
  y : Inport  Port=2
  Calc Carry : Logic  AllPortsSameDT=off  OutDataTypeStr=boolean
  Calc Sum : Logic  Operator=XOR  AllPortsSameDT=off  OutDataTypeStr=boolean
  C : Outport
  S : Outport  Port=2
  wires:
  Calc Carry/1 -> C/1
  x/1 -> Calc Carry/1, Calc Sum/1
  Calc Sum/1 -> S/1
  y/1 -> Calc Sum/2, Calc Carry/2

== system labFinal_3/8-bit Multiply/Half_Adder8 ==
  x : Inport
  y : Inport  Port=2
  Calc Carry : Logic  AllPortsSameDT=off  OutDataTypeStr=boolean
  Calc Sum : Logic  Operator=XOR  AllPortsSameDT=off  OutDataTypeStr=boolean
  C : Outport
  S : Outport  Port=2
  wires:
  Calc Carry/1 -> C/1
  x/1 -> Calc Carry/1, Calc Sum/1
  Calc Sum/1 -> S/1
  y/1 -> Calc Sum/2, Calc Carry/2

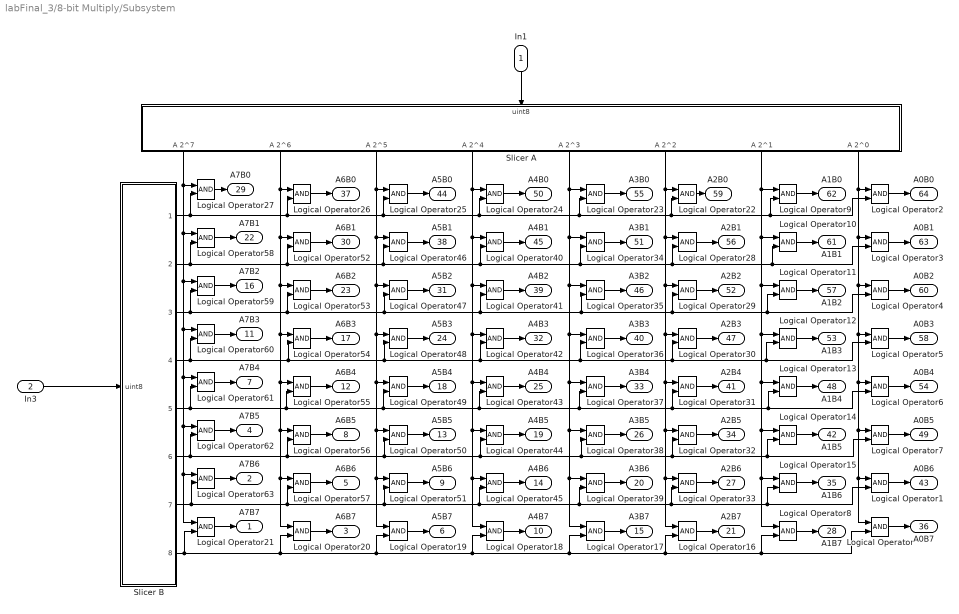
== system labFinal_3/8-bit Multiply/Subsystem ==
  In1 : Inport
  In3 : Inport  Port=2
  Logical Operator{,1..63} (64 alike) : Logic  AllPortsSameDT=off  OutDataTypeStr=boolean
  Slicer A : Subsystem
  Slicer B : Subsystem
  A7B7 : Outport
  A7B6 : Outport  Port=2
  A6B7 : Outport  Port=3
  A7B5 : Outport  Port=4
  A6B6 : Outport  Port=5
  A5B7 : Outport  Port=6
  A7B4 : Outport  Port=7
  A6B5 : Outport  Port=8
  A5B6 : Outport  Port=9
  A4B7 : Outport  Port=10
  A7B3 : Outport  Port=11
  A6B4 : Outport  Port=12
  A5B5 : Outport  Port=13
  A4B6 : Outport  Port=14
  A3B7 : Outport  Port=15
  A7B2 : Outport  Port=16
  A6B3 : Outport  Port=17
  A5B4 : Outport  Port=18
  A4B5 : Outport  Port=19
  A3B6 : Outport  Port=20
  A2B7 : Outport  Port=21
  A7B1 : Outport  Port=22
  A6B2 : Outport  Port=23
  A5B3 : Outport  Port=24
  A4B4 : Outport  Port=25
  A3B5 : Outport  Port=26
  A2B6 : Outport  Port=27
  A1B7 : Outport  Port=28
  A7B0 : Outport  Port=29
  A6B1 : Outport  Port=30
  A5B2 : Outport  Port=31
  A4B3 : Outport  Port=32
  A3B4 : Outport  Port=33
  A2B5 : Outport  Port=34
  A1B6 : Outport  Port=35
  A0B7 : Outport  Port=36
  A6B0 : Outport  Port=37
  A5B1 : Outport  Port=38
  A4B2 : Outport  Port=39
  A3B3 : Outport  Port=40
  A2B4 : Outport  Port=41
  A1B5 : Outport  Port=42
  A0B6 : Outport  Port=43
  A5B0 : Outport  Port=44
  A4B1 : Outport  Port=45
  A3B2 : Outport  Port=46
  A2B3 : Outport  Port=47
  A1B4 : Outport  Port=48
  A0B5 : Outport  Port=49
  A4B0 : Outport  Port=50
  A3B1 : Outport  Port=51
  A2B2 : Outport  Port=52
  A1B3 : Outport  Port=53
  A0B4 : Outport  Port=54
  A3B0 : Outport  Port=55
  A2B1 : Outport  Port=56
  A1B2 : Outport  Port=57
  A0B3 : Outport  Port=58
  A2B0 : Outport  Port=59
  A0B2 : Outport  Port=60
  A1B1 : Outport  Port=61
  A1B0 : Outport  Port=62
  A0B1 : Outport  Port=63
  A0B0 : Outport  Port=64
  wires:
  Logical Operator48/1 -> A5B3/1
  Logical Operator41/1 -> A4B2/1
  Logical Operator49/1 -> A5B4/1
  Logical Operator23/1 -> A3B0/1
  Logical Operator46/1 -> A5B1/1
  Logical Operator21/1 -> A7B7/1
  Logical Operator26/1 -> A6B0/1
  Logical Operator/1 -> A0B7/1
  Logical Operator43/1 -> A4B4/1
  Logical Operator42/1 -> A4B3/1
  Logical Operator32/1 -> A2B5/1
  Logical Operator5/1 -> A0B3/1
  Logical Operator56/1 -> A6B5/1
  Logical Operator37/1 -> A3B4/1
  Logical Operator50/1 -> A5B5/1
  Logical Operator57/1 -> A6B6/1
  Logical Operator29/1 -> A2B2/1
  Logical Operator39/1 -> A3B6/1
  Slicer B/3(B 2^2) -> Logical Operator59/2, Logical Operator53/2, Logical Operator47/2, Logical Operator41/2, Logical Operator35/2, Logical Operator4/2, Logical Operator11/2, Logical Operator29/2
  Logical Operator1/1 -> A0B6/1
  Logical Operator11/1 -> A1B2/1
  Logical Operator15/1 -> A1B6/1
  Logical Operator47/1 -> A5B2/1
  Slicer B/7(B 2^6) -> Logical Operator63/2, Logical Operator57/2, Logical Operator51/2, Logical Operator45/2, Logical Operator39/2, Logical Operator1/2, Logical Operator15/2, Logical Operator33/2
  Slicer B/5(B 2^4) -> Logical Operator61/2, Logical Operator55/2, Logical Operator49/2, Logical Operator43/2, Logical Operator37/2, Logical Operator6/2, Logical Operator13/2, Logical Operator31/2
  Logical Operator18/1 -> A4B7/1
  Slicer A/3(A 2^5) -> Logical Operator25/1, Logical Operator46/1, Logical Operator47/1, Logical Operator48/1, Logical Operator49/1, Logical Operator50/1, Logical Operator51/1, Logical Operator19/1
  Logical Operator53/1 -> A6B2/1
  Logical Operator55/1 -> A6B4/1
  Logical Operator58/1 -> A7B1/1
  Logical Operator25/1 -> A5B0/1
  Logical Operator59/1 -> A7B2/1
  Logical Operator63/1 -> A7B6/1
  In3/1 -> Slicer B/1(uint8)
  Logical Operator6/1 -> A0B4/1
  Logical Operator4/1 -> A0B2/1
  Slicer B/2(B 2^1) -> Logical Operator58/2, Logical Operator52/2, Logical Operator46/2, Logical Operator40/2, Logical Operator34/2, Logical Operator3/2, Logical Operator10/2, Logical Operator28/2
  Logical Operator12/1 -> A1B3/1
  Logical Operator34/1 -> A3B1/1
  Logical Operator60/1 -> A7B3/1
  Logical Operator31/1 -> A2B4/1
  Logical Operator10/1 -> A1B1/1
  Logical Operator36/1 -> A3B3/1
  Logical Operator35/1 -> A3B2/1
  Logical Operator44/1 -> A4B5/1
  Logical Operator62/1 -> A7B5/1
  Logical Operator51/1 -> A5B6/1
  Slicer A/1(A 2^7) -> Logical Operator27/1, Logical Operator58/1, Logical Operator59/1, Logical Operator60/1, Logical Operator61/1, Logical Operator62/1, Logical Operator63/1, Logical Operator21/1
  Logical Operator24/1 -> A4B0/1
  Logical Operator33/1 -> A2B6/1
  Slicer B/8(B 2^7) -> Logical Operator21/2, Logical Operator20/2, Logical Operator19/2, Logical Operator18/2, Logical Operator17/2, Logical Operator16/2, Logical Operator/2, Logical Operator8/2
  Logical Operator40/1 -> A4B1/1
  Slicer A/6(A 2^2) -> Logical Operator22/1, Logical Operator28/1, Logical Operator29/1, Logical Operator30/1, Logical Operator31/1, Logical Operator32/1, Logical Operator33/1, Logical Operator16/1
  Logical Operator20/1 -> A6B7/1
  Logical Operator3/1 -> A0B1/1
  Logical Operator22/1 -> A2B0/1
  Logical Operator45/1 -> A4B6/1
  Slicer A/4(A 2^4) -> Logical Operator24/1, Logical Operator40/1, Logical Operator41/1, Logical Operator42/1, Logical Operator43/1, Logical Operator44/1, Logical Operator45/1, Logical Operator18/1
  Logical Operator17/1 -> A3B7/1
  Logical Operator30/1 -> A2B3/1
  Logical Operator8/1 -> A1B7/1
  Logical Operator38/1 -> A3B5/1
  Logical Operator13/1 -> A1B4/1
  Logical Operator7/1 -> A0B5/1
  Logical Operator16/1 -> A2B7/1
  Slicer B/1("B 2^0 ") -> Logical Operator26/2, Logical Operator25/2, Logical Operator2/2, Logical Operator9/2, Logical Operator22/2, Logical Operator23/2, Logical Operator24/2, Logical Operator27/2
  Slicer A/8("A 2^0 ") -> Logical Operator2/1, Logical Operator3/1, Logical Operator4/1, Logical Operator5/1, Logical Operator6/1, Logical Operator7/1, Logical Operator1/1, Logical Operator/1
  Logical Operator54/1 -> A6B3/1
  Slicer A/7(A 2^1) -> Logical Operator10/1, Logical Operator11/1, Logical Operator12/1, Logical Operator13/1, Logical Operator14/1, Logical Operator15/1, Logical Operator8/1, Logical Operator9/1
  Logical Operator19/1 -> A5B7/1
  Slicer A/5(A 2^3) -> Logical Operator23/1, Logical Operator34/1, Logical Operator35/1, Logical Operator36/1, Logical Operator37/1, Logical Operator38/1, Logical Operator39/1, Logical Operator17/1
  Logical Operator2/1 -> A0B0/1
  Slicer B/6(B 2^5) -> Logical Operator62/2, Logical Operator56/2, Logical Operator50/2, Logical Operator44/2, Logical Operator7/2, Logical Operator14/2, Logical Operator32/2, Logical Operator38/2
  Logical Operator28/1 -> A2B1/1
  Slicer B/4(B 2^3) -> Logical Operator60/2, Logical Operator54/2, Logical Operator48/2, Logical Operator42/2, Logical Operator36/2, Logical Operator5/2, Logical Operator12/2, Logical Operator30/2
  Logical Operator61/1 -> A7B4/1
  Logical Operator52/1 -> A6B1/1
  In1/1 -> Slicer A/1(uint8)
  Logical Operator14/1 -> A1B5/1
  Logical Operator27/1 -> A7B0/1
  Logical Operator9/1 -> A1B0/1
  Slicer A/2(A 2^6) -> Logical Operator26/1, Logical Operator52/1, Logical Operator53/1, Logical Operator54/1, Logical Operator55/1, Logical Operator56/1, Logical Operator57/1, Logical Operator20/1

== system labFinal_3/8-bit Multiply/2^1/Half_Adder ==
  x : Inport
  y : Inport  Port=2
  Calc Carry : Logic  AllPortsSameDT=off  OutDataTypeStr=boolean
  Calc Sum : Logic  Operator=XOR  AllPortsSameDT=off  OutDataTypeStr=boolean
  Sum : Outport
  Carry : Outport  Port=2
  wires:
  Calc Carry/1 -> Carry/1
  x/1 -> Calc Carry/1, Calc Sum/1
  Calc Sum/1 -> Sum/1
  y/1 -> Calc Sum/2, Calc Carry/2

== system labFinal_3/8-bit Multiply/2^1/Half_Adder1 ==
  x : Inport
  y : Inport  Port=2
  Calc Carry : Logic  AllPortsSameDT=off  OutDataTypeStr=boolean
  Calc Sum : Logic  Operator=XOR  AllPortsSameDT=off  OutDataTypeStr=boolean
  Sum : Outport
  Carry : Outport  Port=2
  wires:
  Calc Carry/1 -> Carry/1
  x/1 -> Calc Carry/1, Calc Sum/1
  Calc Sum/1 -> Sum/1
  y/1 -> Calc Sum/2, Calc Carry/2

== system labFinal_3/8-bit Multiply/2^10/Half_Adder ==
  x : Inport
  y : Inport  Port=2
  Calc Carry : Logic  AllPortsSameDT=off  OutDataTypeStr=boolean
  Calc Sum : Logic  Operator=XOR  AllPortsSameDT=off  OutDataTypeStr=boolean
  Sum : Outport
  Carry : Outport  Port=2
  wires:
  Calc Carry/1 -> Carry/1
  x/1 -> Calc Carry/1, Calc Sum/1
  Calc Sum/1 -> Sum/1
  y/1 -> Calc Sum/2, Calc Carry/2

== system labFinal_3/8-bit Multiply/2^10/Half_Adder1 ==
  x : Inport
  y : Inport  Port=2
  Calc Carry : Logic  AllPortsSameDT=off  OutDataTypeStr=boolean
  Calc Sum : Logic  Operator=XOR  AllPortsSameDT=off  OutDataTypeStr=boolean
  Sum : Outport
  Carry : Outport  Port=2
  wires:
  Calc Carry/1 -> Carry/1
  x/1 -> Calc Carry/1, Calc Sum/1
  Calc Sum/1 -> Sum/1
  y/1 -> Calc Sum/2, Calc Carry/2

== system labFinal_3/8-bit Multiply/2^11/Half_Adder ==
  x : Inport
  y : Inport  Port=2
  Calc Carry : Logic  AllPortsSameDT=off  OutDataTypeStr=boolean
  Calc Sum : Logic  Operator=XOR  AllPortsSameDT=off  OutDataTypeStr=boolean
  Sum : Outport
  Carry : Outport  Port=2
  wires:
  Calc Carry/1 -> Carry/1
  x/1 -> Calc Carry/1, Calc Sum/1
  Calc Sum/1 -> Sum/1
  y/1 -> Calc Sum/2, Calc Carry/2

== system labFinal_3/8-bit Multiply/2^11/Half_Adder1 ==
  x : Inport
  y : Inport  Port=2
  Calc Carry : Logic  AllPortsSameDT=off  OutDataTypeStr=boolean
  Calc Sum : Logic  Operator=XOR  AllPortsSameDT=off  OutDataTypeStr=boolean
  Sum : Outport
  Carry : Outport  Port=2
  wires:
  Calc Carry/1 -> Carry/1
  x/1 -> Calc Carry/1, Calc Sum/1
  Calc Sum/1 -> Sum/1
  y/1 -> Calc Sum/2, Calc Carry/2

== system labFinal_3/8-bit Multiply/2^12/Half_Adder ==
  x : Inport
  y : Inport  Port=2
  Calc Carry : Logic  AllPortsSameDT=off  OutDataTypeStr=boolean
  Calc Sum : Logic  Operator=XOR  AllPortsSameDT=off  OutDataTypeStr=boolean
  Sum : Outport
  Carry : Outport  Port=2
  wires:
  Calc Carry/1 -> Carry/1
  x/1 -> Calc Carry/1, Calc Sum/1
  Calc Sum/1 -> Sum/1
  y/1 -> Calc Sum/2, Calc Carry/2

== system labFinal_3/8-bit Multiply/2^12/Half_Adder1 ==
  x : Inport
  y : Inport  Port=2
  Calc Carry : Logic  AllPortsSameDT=off  OutDataTypeStr=boolean
  Calc Sum : Logic  Operator=XOR  AllPortsSameDT=off  OutDataTypeStr=boolean
  Sum : Outport
  Carry : Outport  Port=2
  wires:
  Calc Carry/1 -> Carry/1
  x/1 -> Calc Carry/1, Calc Sum/1
  Calc Sum/1 -> Sum/1
  y/1 -> Calc Sum/2, Calc Carry/2

== system labFinal_3/8-bit Multiply/2^13/Half_Adder ==
  x : Inport
  y : Inport  Port=2
  Calc Carry : Logic  AllPortsSameDT=off  OutDataTypeStr=boolean
  Calc Sum : Logic  Operator=XOR  AllPortsSameDT=off  OutDataTypeStr=boolean
  Sum : Outport
  Carry : Outport  Port=2
  wires:
  Calc Carry/1 -> Carry/1
  x/1 -> Calc Carry/1, Calc Sum/1
  Calc Sum/1 -> Sum/1
  y/1 -> Calc Sum/2, Calc Carry/2

== system labFinal_3/8-bit Multiply/2^13/Half_Adder1 ==
  x : Inport
  y : Inport  Port=2
  Calc Carry : Logic  AllPortsSameDT=off  OutDataTypeStr=boolean
  Calc Sum : Logic  Operator=XOR  AllPortsSameDT=off  OutDataTypeStr=boolean
  Sum : Outport
  Carry : Outport  Port=2
  wires:
  Calc Carry/1 -> Carry/1
  x/1 -> Calc Carry/1, Calc Sum/1
  Calc Sum/1 -> Sum/1
  y/1 -> Calc Sum/2, Calc Carry/2

== system labFinal_3/8-bit Multiply/2^14/Half_Adder ==
  x : Inport
  y : Inport  Port=2
  Calc Carry : Logic  AllPortsSameDT=off  OutDataTypeStr=boolean
  Calc Sum : Logic  Operator=XOR  AllPortsSameDT=off  OutDataTypeStr=boolean
  Sum : Outport
  Carry : Outport  Port=2
  wires:
  Calc Carry/1 -> Carry/1
  x/1 -> Calc Carry/1, Calc Sum/1
  Calc Sum/1 -> Sum/1
  y/1 -> Calc Sum/2, Calc Carry/2

== system labFinal_3/8-bit Multiply/2^14/Half_Adder1 ==
  x : Inport
  y : Inport  Port=2
  Calc Carry : Logic  AllPortsSameDT=off  OutDataTypeStr=boolean
  Calc Sum : Logic  Operator=XOR  AllPortsSameDT=off  OutDataTypeStr=boolean
  Sum : Outport
  Carry : Outport  Port=2
  wires:
  Calc Carry/1 -> Carry/1
  x/1 -> Calc Carry/1, Calc Sum/1
  Calc Sum/1 -> Sum/1
  y/1 -> Calc Sum/2, Calc Carry/2

== system labFinal_3/8-bit Multiply/2^15/Half_Adder ==
  x : Inport
  y : Inport  Port=2
  Calc Carry : Logic  AllPortsSameDT=off  OutDataTypeStr=boolean
  Calc Sum : Logic  Operator=XOR  AllPortsSameDT=off  OutDataTypeStr=boolean
  Sum : Outport
  Carry : Outport  Port=2
  wires:
  Calc Carry/1 -> Carry/1
  x/1 -> Calc Carry/1, Calc Sum/1
  Calc Sum/1 -> Sum/1
  y/1 -> Calc Sum/2, Calc Carry/2

== system labFinal_3/8-bit Multiply/2^15/Half_Adder1 ==
  x : Inport
  y : Inport  Port=2
  Calc Carry : Logic  AllPortsSameDT=off  OutDataTypeStr=boolean
  Calc Sum : Logic  Operator=XOR  AllPortsSameDT=off  OutDataTypeStr=boolean
  Sum : Outport
  Carry : Outport  Port=2
  wires:
  Calc Carry/1 -> Carry/1
  x/1 -> Calc Carry/1, Calc Sum/1
  Calc Sum/1 -> Sum/1
  y/1 -> Calc Sum/2, Calc Carry/2

== system labFinal_3/8-bit Multiply/2^16/Half_Adder ==
  x : Inport
  y : Inport  Port=2
  Calc Carry : Logic  AllPortsSameDT=off  OutDataTypeStr=boolean
  Calc Sum : Logic  Operator=XOR  AllPortsSameDT=off  OutDataTypeStr=boolean
  Sum : Outport
  Carry : Outport  Port=2
  wires:
  Calc Carry/1 -> Carry/1
  x/1 -> Calc Carry/1, Calc Sum/1
  Calc Sum/1 -> Sum/1
  y/1 -> Calc Sum/2, Calc Carry/2

== system labFinal_3/8-bit Multiply/2^16/Half_Adder1 ==
  x : Inport
  y : Inport  Port=2
  Calc Carry : Logic  AllPortsSameDT=off  OutDataTypeStr=boolean
  Calc Sum : Logic  Operator=XOR  AllPortsSameDT=off  OutDataTypeStr=boolean
  Sum : Outport
  Carry : Outport  Port=2
  wires:
  Calc Carry/1 -> Carry/1
  x/1 -> Calc Carry/1, Calc Sum/1
  Calc Sum/1 -> Sum/1
  y/1 -> Calc Sum/2, Calc Carry/2

== system labFinal_3/8-bit Multiply/2^17/Half_Adder ==
  x : Inport
  y : Inport  Port=2
  Calc Carry : Logic  AllPortsSameDT=off  OutDataTypeStr=boolean
  Calc Sum : Logic  Operator=XOR  AllPortsSameDT=off  OutDataTypeStr=boolean
  Sum : Outport
  Carry : Outport  Port=2
  wires:
  Calc Carry/1 -> Carry/1
  x/1 -> Calc Carry/1, Calc Sum/1
  Calc Sum/1 -> Sum/1
  y/1 -> Calc Sum/2, Calc Carry/2

== system labFinal_3/8-bit Multiply/2^17/Half_Adder1 ==
  x : Inport
  y : Inport  Port=2
  Calc Carry : Logic  AllPortsSameDT=off  OutDataTypeStr=boolean
  Calc Sum : Logic  Operator=XOR  AllPortsSameDT=off  OutDataTypeStr=boolean
  Sum : Outport
  Carry : Outport  Port=2
  wires:
  Calc Carry/1 -> Carry/1
  x/1 -> Calc Carry/1, Calc Sum/1
  Calc Sum/1 -> Sum/1
  y/1 -> Calc Sum/2, Calc Carry/2

== system labFinal_3/8-bit Multiply/2^18/Half_Adder ==
  x : Inport
  y : Inport  Port=2
  Calc Carry : Logic  AllPortsSameDT=off  OutDataTypeStr=boolean
  Calc Sum : Logic  Operator=XOR  AllPortsSameDT=off  OutDataTypeStr=boolean
  Sum : Outport
  Carry : Outport  Port=2
  wires:
  Calc Carry/1 -> Carry/1
  x/1 -> Calc Carry/1, Calc Sum/1
  Calc Sum/1 -> Sum/1
  y/1 -> Calc Sum/2, Calc Carry/2

== system labFinal_3/8-bit Multiply/2^18/Half_Adder1 ==
  x : Inport
  y : Inport  Port=2
  Calc Carry : Logic  AllPortsSameDT=off  OutDataTypeStr=boolean
  Calc Sum : Logic  Operator=XOR  AllPortsSameDT=off  OutDataTypeStr=boolean
  Sum : Outport
  Carry : Outport  Port=2
  wires:
  Calc Carry/1 -> Carry/1
  x/1 -> Calc Carry/1, Calc Sum/1
  Calc Sum/1 -> Sum/1
  y/1 -> Calc Sum/2, Calc Carry/2

== system labFinal_3/8-bit Multiply/2^19/Half_Adder ==
  x : Inport
  y : Inport  Port=2
  Calc Carry : Logic  AllPortsSameDT=off  OutDataTypeStr=boolean
  Calc Sum : Logic  Operator=XOR  AllPortsSameDT=off  OutDataTypeStr=boolean
  Sum : Outport
  Carry : Outport  Port=2
  wires:
  Calc Carry/1 -> Carry/1
  x/1 -> Calc Carry/1, Calc Sum/1
  Calc Sum/1 -> Sum/1
  y/1 -> Calc Sum/2, Calc Carry/2

== system labFinal_3/8-bit Multiply/2^19/Half_Adder1 ==
  x : Inport
  y : Inport  Port=2
  Calc Carry : Logic  AllPortsSameDT=off  OutDataTypeStr=boolean
  Calc Sum : Logic  Operator=XOR  AllPortsSameDT=off  OutDataTypeStr=boolean
  Sum : Outport
  Carry : Outport  Port=2
  wires:
  Calc Carry/1 -> Carry/1
  x/1 -> Calc Carry/1, Calc Sum/1
  Calc Sum/1 -> Sum/1
  y/1 -> Calc Sum/2, Calc Carry/2

== system labFinal_3/8-bit Multiply/2^2/Half_Adder ==
  x : Inport
  y : Inport  Port=2
  Calc Carry : Logic  AllPortsSameDT=off  OutDataTypeStr=boolean
  Calc Sum : Logic  Operator=XOR  AllPortsSameDT=off  OutDataTypeStr=boolean
  Sum : Outport
  Carry : Outport  Port=2
  wires:
  Calc Carry/1 -> Carry/1
  x/1 -> Calc Carry/1, Calc Sum/1
  Calc Sum/1 -> Sum/1
  y/1 -> Calc Sum/2, Calc Carry/2

== system labFinal_3/8-bit Multiply/2^2/Half_Adder1 ==
  x : Inport
  y : Inport  Port=2
  Calc Carry : Logic  AllPortsSameDT=off  OutDataTypeStr=boolean
  Calc Sum : Logic  Operator=XOR  AllPortsSameDT=off  OutDataTypeStr=boolean
  Sum : Outport
  Carry : Outport  Port=2
  wires:
  Calc Carry/1 -> Carry/1
  x/1 -> Calc Carry/1, Calc Sum/1
  Calc Sum/1 -> Sum/1
  y/1 -> Calc Sum/2, Calc Carry/2

== system labFinal_3/8-bit Multiply/2^20/Half_Adder ==
  x : Inport
  y : Inport  Port=2
  Calc Carry : Logic  AllPortsSameDT=off  OutDataTypeStr=boolean
  Calc Sum : Logic  Operator=XOR  AllPortsSameDT=off  OutDataTypeStr=boolean
  Sum : Outport
  Carry : Outport  Port=2
  wires:
  Calc Carry/1 -> Carry/1
  x/1 -> Calc Carry/1, Calc Sum/1
  Calc Sum/1 -> Sum/1
  y/1 -> Calc Sum/2, Calc Carry/2

== system labFinal_3/8-bit Multiply/2^20/Half_Adder1 ==
  x : Inport
  y : Inport  Port=2
  Calc Carry : Logic  AllPortsSameDT=off  OutDataTypeStr=boolean
  Calc Sum : Logic  Operator=XOR  AllPortsSameDT=off  OutDataTypeStr=boolean
  Sum : Outport
  Carry : Outport  Port=2
  wires:
  Calc Carry/1 -> Carry/1
  x/1 -> Calc Carry/1, Calc Sum/1
  Calc Sum/1 -> Sum/1
  y/1 -> Calc Sum/2, Calc Carry/2

== system labFinal_3/8-bit Multiply/2^21/Half_Adder ==
  x : Inport
  y : Inport  Port=2
  Calc Carry : Logic  AllPortsSameDT=off  OutDataTypeStr=boolean
  Calc Sum : Logic  Operator=XOR  AllPortsSameDT=off  OutDataTypeStr=boolean
  Sum : Outport
  Carry : Outport  Port=2
  wires:
  Calc Carry/1 -> Carry/1
  x/1 -> Calc Carry/1, Calc Sum/1
  Calc Sum/1 -> Sum/1
  y/1 -> Calc Sum/2, Calc Carry/2

== system labFinal_3/8-bit Multiply/2^21/Half_Adder1 ==
  x : Inport
  y : Inport  Port=2
  Calc Carry : Logic  AllPortsSameDT=off  OutDataTypeStr=boolean
  Calc Sum : Logic  Operator=XOR  AllPortsSameDT=off  OutDataTypeStr=boolean
  Sum : Outport
  Carry : Outport  Port=2
  wires:
  Calc Carry/1 -> Carry/1
  x/1 -> Calc Carry/1, Calc Sum/1
  Calc Sum/1 -> Sum/1
  y/1 -> Calc Sum/2, Calc Carry/2

== system labFinal_3/8-bit Multiply/2^22/Half_Adder ==
  x : Inport
  y : Inport  Port=2
  Calc Carry : Logic  AllPortsSameDT=off  OutDataTypeStr=boolean
  Calc Sum : Logic  Operator=XOR  AllPortsSameDT=off  OutDataTypeStr=boolean
  Sum : Outport
  Carry : Outport  Port=2
  wires:
  Calc Carry/1 -> Carry/1
  x/1 -> Calc Carry/1, Calc Sum/1
  Calc Sum/1 -> Sum/1
  y/1 -> Calc Sum/2, Calc Carry/2
